simulink model "ladder_filter"  (Simulink 6.0)
settings: Solver=ode45  StartTime=0.0  StopTime=10.0  RelTol=1e-3
undefined symbols (not defined in the file or in its folder): Fs
libraries: rfports1 x4, rfladderfilters1 x2, dspsnks4 x1, simulink x1, dspsrcs4 x1
settings Model: Creator=ashivapr  LastModifiedBy=rzeng  ProdHWDeviceType=Specified  UpdateModelReferenceTargets=IfOutOfDate
settings DataIOCC: SaveOutput=off  SaveTime=off  SignalLoggingName=logsOut
settings DebuggingCC: CheckExecutionContextPreStartOutputMsg=on  CheckExecutionContextRuntimeOutputMsg=on  SolverPrmCheckMsg=none
settings HardwareCC: ProdHWDeviceType=Specified
settings ModelReferenceCC: UpdateModelReferenceTargets=IfOutOfDate
settings GRTTargetCC: UtilityFuncGeneration=Automatic  LifeSpan=inf
settings SFSimCC: SFSimApplyToAllLibs=on  SFSimBuildMode=Incremental

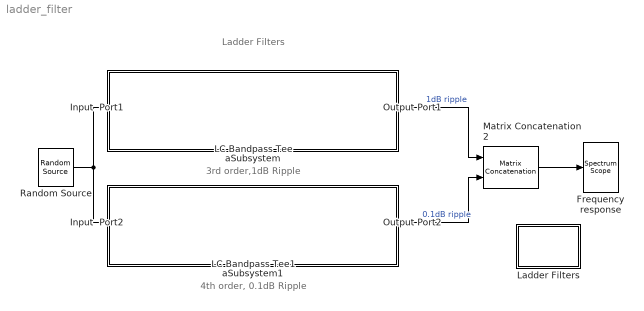
== system ladder_filter ==
  note: 3rd order,1dB Ripple
  note: 4th order, 0.1dB Ripple
  note: Ladder Filters
  Frequency response : dspsnks4/Spectrum Scope  ScopeProperties=off  Domain=Frequency  HorizSpan=1  UseBuffer=off  BufferSize=128  Overlap=64  inpFftLenInherit=off  FFTlength=1024  numAvg=400  DisplayProperties=off  AxisGrid=on  Memory=off  FrameNumber=off  AxisLegend=on  AxisZoom=off  OpenScopeAtSimStart=on  OpenScopeImmediately=off  FigPos=[8 379 666 232]  AxisProperties=on  XUnits=Hertz  XRange=[-Fs/2...Fs/2]  InheritXIncr=on  XIncr=1.0  XLabel=Samples  YUnits=dB  YLabel=Magnitude, dB  LineProperties=off  LineColors=[0 0 1]|[1 0 0]
      settings: YMin=-21.735349676775  YMax=1.75497648078704
  Input  Port1 : rfports1/Input Port  Description=source block  MaxLength=128  Fc=75e6  Ts=1e-7  Zs=0.01  NoiseFlag=off  seed=67987  GoToTag=ABBAABCAFAMDPCMLJHTPGDV
  Input  Port2 : rfports1/Input Port  Description=source block  MaxLength=128  Fc=75e6  Ts=1e-7  Zs=0.01  NoiseFlag=off  seed=67987  GoToTag=BCCBBCDBGBNEQDNMKIUQHEW
  LC Bandpass Tee : rfladderfilters1/LC Bandpass Tee  PhysicalDomain=rfsystemsdomain  SubClassName=lcbandpasstee  LeftPortType=p1  RightPortType=p1  LConnTagsString=__newl0  RConnTagsString=__newr0  L="[0.0037561  1.3566e-005    0.0025192]"  C="[1.1989e-015  3.3195e-013  1.7875e-015]"  DisplayData=off  PlotFreq=Derived from Input Port parameters  PlotFreqNoSim=User specified  Freq=[70e6:1.0e5:80e6]  AllPlotType=X-Y plane  NetworkData=S21  SmithData=S11  PolarData=S11  ComplexFormat=Magnitude (decibels)  DBFormat=Magnitude (decibels)  NoneFormat=None
  LC Bandpass Tee1 : rfladderfilters1/LC Bandpass Tee  PhysicalDomain=rfsystemsdomain  SubClassName=lcbandpasstee  LeftPortType=p1  RightPortType=p1  LConnTagsString=__newl0  RConnTagsString=__newr0  L="[0.0034355  1.1202e-005    0.0033081  2.9429e-005]"  C="[1.3108e-015  4.0198e-013  1.3612e-015  1.5302e-013]"  DisplayData=off  PlotFreq=Derived from Input Port parameters  PlotFreqNoSim=User specified  Freq=[70e6:1.0e5:80e6]  AllPlotType=X-Y plane  NetworkData=S21  SmithData=S11  PolarData=S12  ComplexFormat=Magnitude (decibels)  DBFormat=Magnitude (decibels)  NoneFormat=None
  Ladder Filters : Subsystem  EnableExecutionContextPropagation=on
      mask Display: disp('Info')
  Matrix Concatenation2 : simulink/Math Operations/Matrix Concatenation  numInports=2  catMethod=Horizontal
  Output Port1 : rfports1/Output Port  Zl=1e5  num_Models=1  GoToTag=ABBAABCAFAMDPCMLJHTPGDV  DisplayData=off  PlotFreq=Derived from Input Port parameters  Freq=1e9:1e8:3e9  AllPlotType=Composite data  NoBudgetPlot=Composite data  NetworkData=S11  SmithData=S11  PolarData=S11  ComplexFormat=Magnitude (decibels)  DBFormat=Magnitude (decibels)  DBMFormat=dBm  NoneFormat=None
  Output Port2 : rfports1/Output Port  Zl=1e5  num_Models=1  GoToTag=BCCBBCDBGBNEQDNMKIUQHEW  DisplayData=off  PlotFreq=Derived from Input Port parameters  Freq=1e9:1e8:3e9  AllPlotType=Composite data  NoBudgetPlot=Composite data  NetworkData=S11  SmithData=S11  PolarData=S11  ComplexFormat=Magnitude (decibels)  DBFormat=Magnitude (decibels)  DBMFormat=dBm  NoneFormat=None
  Random Source : dspsrcs4/Random Source  SrcType=Gaussian  NormMethod=Ziggurat  CltLength=12  Min=0  Max=1  Mean=0  Var=1  RepMode=Not repeatable  Seed=1  Inherit=off  SampMode=Discrete  SampTime=1e-7  SampFrame=256  DataType=Double  OutComplex=Complex
  aSubsystem : Subsystem  EnableExecutionContextPropagation=on
      mask Display: disp('')
  aSubsystem1 : Subsystem  EnableExecutionContextPropagation=on
      mask Display: disp('')
  wires:
  Random Source/1 -> Input  Port1/1, Input  Port2/1
  Output Port1/1 -> Matrix Concatenation2/1  "1dB ripple"
  Matrix Concatenation2/1 -> Frequency response/1
  Output Port2/1 -> Matrix Concatenation2/2  "0.1dB ripple"
  connections:
  Input  Port1/RConn1 -- LC Bandpass Tee/LConn1
  LC Bandpass Tee/RConn1 -- Output Port1/LConn1
  Input  Port2/RConn1 -- LC Bandpass Tee1/LConn1
  LC Bandpass Tee1/RConn1 -- Output Port2/LConn1

== system ladder_filter/Ladder Filters ==
  note: Ladder Filters
  note: This model shows Chebyshev I filters with a passband ripple of
      | 1dB and 0.1dB implemented using LC Bandpass Tee filters
      | from the Ladder Filters sublibrary.
  note: Filter specifications:
      | Center frequency = 75MHz
      | Bandwidth at 3dB = 7MHz
      | Bandwidth at 45dB = 35MHz
      | Source impedance = 0.01 ohms
      |  Load impedance = 1e5 ohms
  note: The frequency responses of the filters clearly show the
      | difference in passband ripples.
  note: To create the above filter with a passband ripple of 1dB, a filter
      | of 3rd order is required. To realize the same filter with a passband
      | ripple of 0.1dB, a filter of 4th order is required.
  note: Reference: Chris Bowick, RF Circuit Design, 1982, pp 65

== system ladder_filter/aSubsystem ==

== system ladder_filter/aSubsystem1 ==
